simulink model "TS_modling_simulation"  (R2020a)
settings: Solver=VariableStepAuto  StartTime=0.0  StopTime=50  RelTol=1e-3
values from neighbouring files (symbols this model uses):
  A1 = [-1 max(z1) ... (first row only)    [TS_modling_script.m]    (also in cart_pend_script.m = [0 1 0 0; -17.31 0 0 0; 0 0 0 1; 1.7312 0 0 0])
  A2 = [-1 max(z1) ... (first row only)    [TS_modling_script.m]    (also in cart_pend_script.m = [0 1 0 0; -14.32 0 0 0; 0 0 0 1; 0.716 0 0 0])
  A3 = [-1 min(z1) ... (first row only)    [TS_modling_script.m]
  A4 = [-1 min(z1) ... (first row only)    [TS_modling_script.m]
  B = [1;1]    [TS_modling_script.m]
  x0 = [-0.7;1]    [TS_modling_script.m]    (also in cart_pend_script.m = [0.6; 0; 0.1; 0])
libraries: fuzblock x4
settings Model: Creator=amine  LastModifiedBy=hp
settings DebuggingCC: SFMachineParentedDataDiag=error

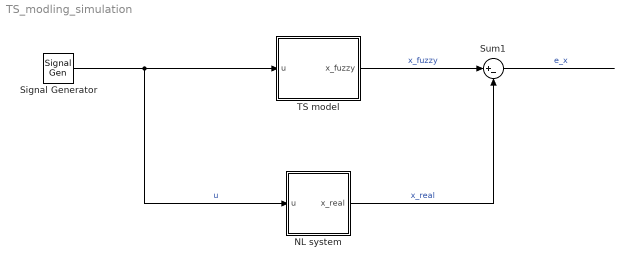
== system TS_modling_simulation ==
  NL system : Subsystem
  Signal Generator : SignalGenerator  WaveForm=square  Amplitude=0.1  Units=rad/sec
  Sum1 : Sum  Inputs=|+-
  TS model : Subsystem
  wires:
  Signal Generator/1 -> TS model/1(u), NL system/1(u)  "u"
  Sum1/1 -> ?  "e_x"
  NL system/1(x_real) -> Sum1/2  "x_real"
  TS model/1(x_fuzzy) -> Sum1/1  "x_fuzzy"

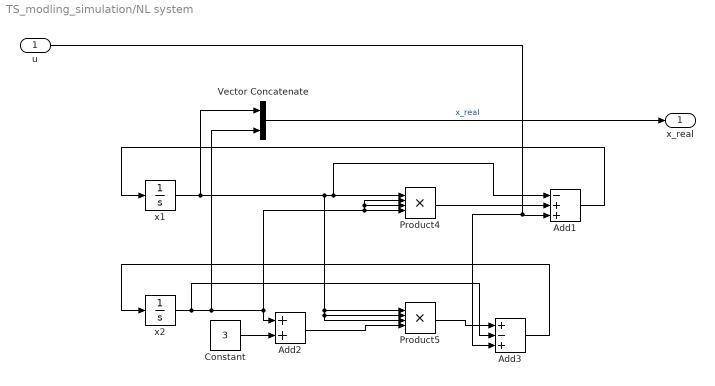
== system TS_modling_simulation/NL system ==
  u : Inport
  Add1 : Sum  Inputs=-++
  Add2 : Sum
  Add3 : Sum  Inputs=+-+
  Constant : Constant  Value=3
  Product4 : Product  Inputs=4
  Product5 : Product  Inputs=4
  Vector Concatenate : Concatenate
  x1 : Integrator  InitialCondition=x0(1)
  x2 : Integrator  InitialCondition=x0(2)
  x_real : Outport
  wires:
  x1/1 -> Vector Concatenate/1, Product5/3, Product5/2, Product5/1, Add1/1, Product4/1
  Add2/1 -> Product5/4
  x2/1 -> Add3/2, Vector Concatenate/2, Add2/1, Product4/3, Product4/2, Product4/4
  Product5/1 -> Add3/1
  Product4/1 -> Add1/2
  Add1/1 -> x1/1
  Constant/1 -> Add2/2
  Add3/1 -> x2/1
  u/1 -> Add3/3, Add1/3
  Vector Concatenate/1 -> x_real/1  "x_real"

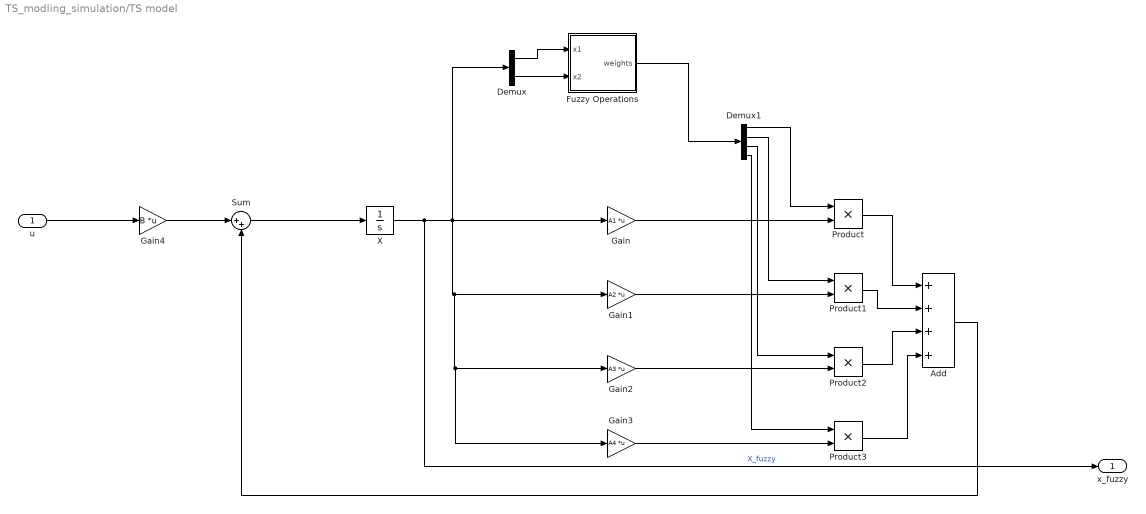
== system TS_modling_simulation/TS model ==
  u : Inport
  Add : Sum  Inputs=++++
  Demux : Demux  Outputs=2
  Demux1 : Demux
  Fuzzy Operations : Subsystem
  Gain : Gain  Gain=A1  Multiplication=Matrix(K*u)
  Gain1 : Gain  Gain=A2  Multiplication=Matrix(K*u)
  Gain2 : Gain  Gain=A3  Multiplication=Matrix(K*u)
  Gain3 : Gain  Gain=A4  Multiplication=Matrix(K*u)
  Gain4 : Gain  Gain=B  Multiplication=Matrix(K*u)
  Product{,1..3} (4 alike) : Product
  Sum : Sum  Inputs=|++
  X : Integrator  InitialCondition=x0
  x_fuzzy : Outport
  wires:
  Product2/1 -> Add/3
  Gain4/1 -> Sum/1
  Fuzzy Operations/1(weights) -> Demux1/1
  Product/1 -> Add/1
  Gain1/1 -> Product1/2
  Product1/1 -> Add/2
  Demux1/2 -> Product1/1
  Sum/1 -> X/1
  X/1 -> x_fuzzy/1, Gain3/1, Gain2/1, Gain1/1, Gain/1, Demux/1  "X_fuzzy"
  Demux1/3 -> Product2/1
  Gain/1 -> Product/2
  Demux/2 -> Fuzzy Operations/2(x2)
  Gain2/1 -> Product2/2
  Add/1 -> Sum/2
  Demux1/1 -> Product/1
  Demux1/4 -> Product3/1
  Demux/1 -> Fuzzy Operations/1(x1)
  Product3/1 -> Add/4
  Gain3/1 -> Product3/2
  u/1 -> Gain4/1

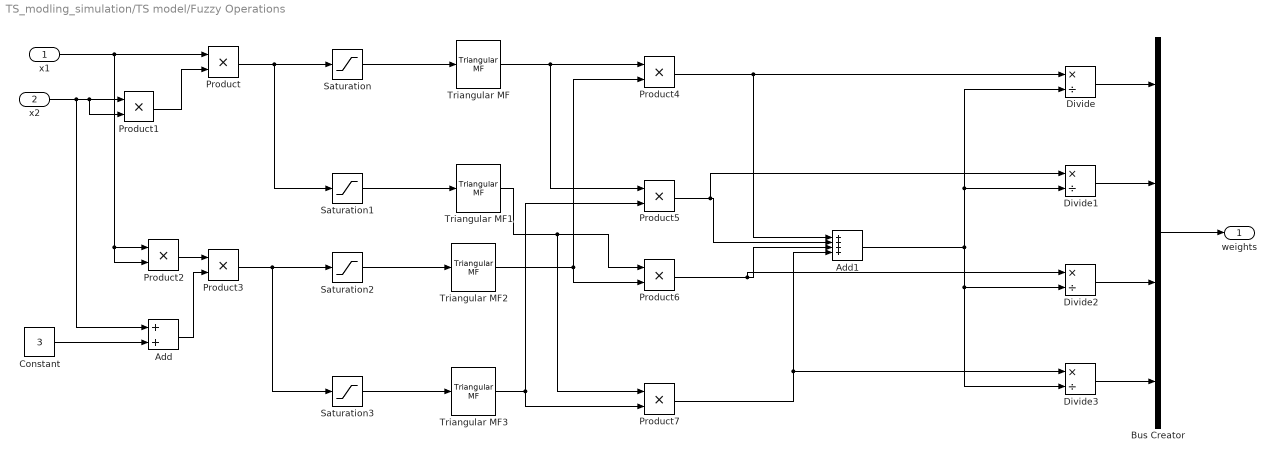
== system TS_modling_simulation/TS model/Fuzzy Operations ==
  x1 : Inport
  x2 : Inport  Port=2
  Add : Sum
  Add1 : Sum  Inputs=++++
  Bus Creator : BusCreator  Inputs=4
  Constant : Constant  Value=3
  Divide{,1..3} (4 alike) : Product  Inputs=*/
  Product{,1..7} (8 alike) : Product
  Saturation{,1..3} (4 alike) : Saturate  UpperLimit=1  LowerLimit=0
  Triangular MF : fuzblock/Membership  Functions/Triangular MF  a=-1  b=1  c=1
      settings: SourceProductBaseCode=FL
  Triangular MF1 : fuzblock/Membership  Functions/Triangular MF  a=-1  b=-1  c=1
      settings: SourceProductBaseCode=FL
  Triangular MF2 : fuzblock/Membership  Functions/Triangular MF  a=0  b=4  c=4
      settings: SourceProductBaseCode=FL
  Triangular MF3 : fuzblock/Membership  Functions/Triangular MF  a=0  b=0  c=4
      settings: SourceProductBaseCode=FL
  weights : Outport
  wires:
  Product6/1 -> Divide2/1, Add1/3
  Triangular MF/1 -> Product5/1, Product4/1
  x2/1 -> Add/1, Product1/2, Product1/1
  x1/1 -> Product2/2, Product2/1, Product/1
  Saturation1/1 -> Triangular MF1/1
  Product4/1 -> Divide/1, Add1/1
  Saturation/1 -> Triangular MF/1
  Product3/1 -> Saturation3/1, Saturation2/1
  Product1/1 -> Product/2
  Triangular MF1/1 -> Product7/1, Product6/1
  Product/1 -> Saturation1/1, Saturation/1
  Saturation3/1 -> Triangular MF3/1
  Triangular MF2/1 -> Product4/2, Product6/2
  Triangular MF3/1 -> Product5/2, Product7/2
  Product7/1 -> Divide3/1, Add1/4
  Constant/1 -> Add/2
  Product5/1 -> Divide1/1, Add1/2
  Bus Creator/1 -> weights/1
  Add/1 -> Product3/2
  Saturation2/1 -> Triangular MF2/1
  Product2/1 -> Product3/1
  Divide/1 -> Bus Creator/1
  Divide1/1 -> Bus Creator/2
  Divide2/1 -> Bus Creator/3
  Divide3/1 -> Bus Creator/4
  Add1/1 -> Divide2/2, Divide3/2, Divide1/2, Divide/2
